simulink subsystem "Inputs_MEGA"  (R2023b)
settings: Solver=VariableStepAuto  StartTime=0.0  StopTime=10.0  RelTol=1e-3
libraries: arduinolib x3
settings Model: Creator=m4ttn  LastModifiedBy=m4ttn
settings RTWCC: GPUComputeCapability=5.0

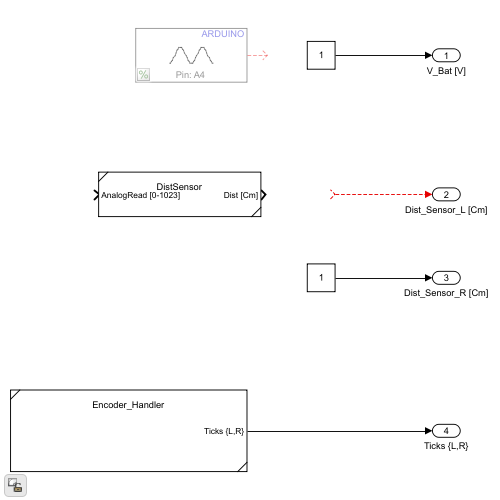
[thumbnail: Simulink's stored preview of the top-level diagram]
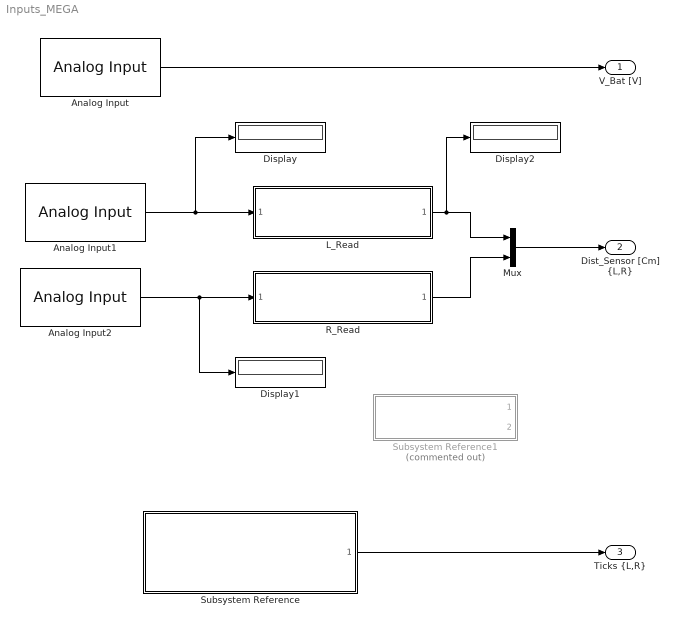
== system Inputs_MEGA ==
  Analog Input : arduinolib/Analog Input  pinNumber=8  ReadResultsOnly=off  ConversionTriggerSource=Software  ExternalTriggerType=uint32( 0 )  OutputDataType=uint16  EnableConversionCompleteNotify=off  EnableOuputStatus=off  SampleTime=-1  blockPlatform=arduino
  Analog Input1 : arduinolib/Analog Input  pinNumber=6  ReadResultsOnly=off  ConversionTriggerSource=Software  ExternalTriggerType=uint32( 0 )  OutputDataType=uint16  EnableConversionCompleteNotify=off  EnableOuputStatus=off  SampleTime=-1  blockPlatform=arduino
  Analog Input2 : arduinolib/Analog Input  pinNumber=7  ReadResultsOnly=off  ConversionTriggerSource=Software  ExternalTriggerType=uint32( 0 )  OutputDataType=uint16  EnableConversionCompleteNotify=off  EnableOuputStatus=off  SampleTime=-1  blockPlatform=arduino
  Display : Display
  Display1 : Display
  Display2 : Display
  L_Read : Subsystem  ReferencedSubsystem=DistSensor
  Mux : Mux  Inputs=2
  R_Read : Subsystem  ReferencedSubsystem=DistSensor
  Subsystem Reference : Subsystem  ReferencedSubsystem=Encoder_Handler
  Subsystem Reference1 : Subsystem  Commented=on  ReferencedSubsystem=VL53X_multipleSensor
  V_Bat [V] : Outport
  "Dist_Sensor [Cm] {L,R}" : Outport  Port=2  OutDataTypeStr=uint8
  "Ticks {L,R}" : Outport  Port=3
  wires:
  Mux/1 -> "Dist_Sensor [Cm] {L,R}"/1
  L_Read/1 -> Mux/1, Display2/1
  R_Read/1 -> Mux/2
  Analog Input1/1 -> L_Read/1, Display/1
  Analog Input2/1 -> R_Read/1, Display1/1
  Subsystem Reference/1 -> "Ticks {L,R}"/1
  Analog Input/1 -> V_Bat [V]/1
